simulink library "boiler"  (R2018a)
settings: Solver=VariableStepAuto  StartTime=0.0  StopTime=10.0  RelTol=1e-3
libraries: fl_lib x4
settings Model: Creator=ChLan  LastModifiedBy=ChLan

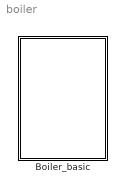
== system boiler ==
  Boiler_basic : Subsystem

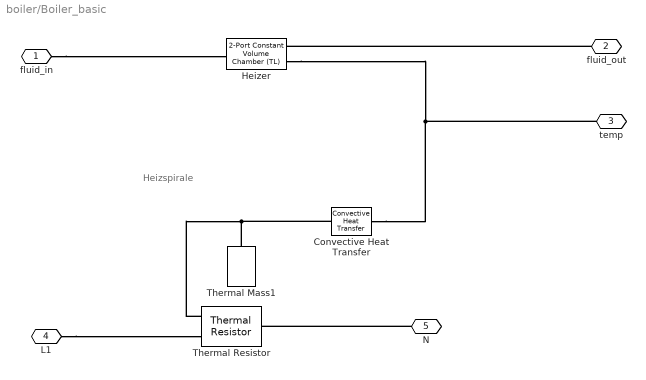
== system boiler/Boiler_basic ==
  note: Heizspirale
  Convective Heat Transfer : fl_lib/Thermal/Thermal Elements/Convective Heat Transfer  area=1000 cm^2  heat_tr_coeff=1000 W/(m^2 * K)  T_specify=off  T_priority=None  T=0 K  T_nominal_specify=off  T_nominal_unit=K  T_nominal_value=1  Q_specify=off  Q_priority=None  Q=0 W  Q_nominal_specify=off  Q_nominal_unit=W  Q_nominal_value=1
  Heizer : fl_lib/Thermal Liquid/Elements/2-Port Constant Volume Chamber (TL)  volume=0.25 l  area_A=0.01 m^2  area_B=0.01 m^2  p_chamber_specify=on  p_chamber_priority=Low  p_chamber=0.101325 MPa  p_chamber_nominal_specify=off  p_chamber_nominal_unit=MPa  p_chamber_nominal_value=1  T_chamber_specify=on  T_chamber_priority=High  T_chamber=300 K  T_chamber_nominal_specify=off  T_chamber_nominal_unit=K  T_chamber_nominal_value=1  u_chamber_specify=off  u_chamber_priority=None  u_chamber=83.90600000000001 kJ/kg  u_chamber_nominal_specify=off  u_chamber_nominal_unit=kJ/kg  u_chamber_nominal_value=1  rho_specify=off  rho_priority=None  rho=998.21 kg/m^3  rho_nominal_specify=off  rho_nominal_unit=kg/m^3  rho_nominal_value=1
      settings: SourceProductName=Simscape  SourceProductBaseCode=SS
  Thermal Mass1 : fl_lib/Thermal/Thermal Elements/Thermal Mass  mass=0.05 kg  sp_heat=447 J/kg/K  T_specify=off  T_priority=High  T=300 K  T_nominal_specify=off  T_nominal_unit=K  T_nominal_value=1  Q_specify=off  Q_priority=None  Q=0 W  Q_nominal_specify=off  Q_nominal_unit=W  Q_nominal_value=1
  Thermal Resistor : fl_lib/Electrical/Electrical Elements/Thermal Resistor  R0=35 Ohm  T0=298.15 K  alpha=50e-6 1/K  tc=10 s  K_d=1e-3 W/K  T_specify=off  T_priority=High  T=300 K  T_nominal_specify=off  T_nominal_unit=K  T_nominal_value=1
      settings: SourceProductName=Simscape  SourceProductBaseCode=SS
  fluid_in : PMIOPort  Side=Left
  fluid_out : PMIOPort  Port=2  Side=Right
  temp : PMIOPort  Port=3  Side=Right
  L1 : PMIOPort  Port=4  Side=Left
  N : PMIOPort  Port=5  Side=Right
  connections:
  fluid_in/RConn1 -- Heizer/RConn1
  fluid_out/RConn1 -- Heizer/LConn1
  N/RConn1 -- Thermal Resistor/RConn1
  Convective Heat Transfer/LConn1 -- Thermal Mass1/LConn1 -- Thermal Resistor/LConn1
  temp/RConn1 -- Heizer/LConn2 -- Convective Heat Transfer/RConn1
  L1/RConn1 -- Thermal Resistor/LConn2
